simulink subsystem "Find_Catmull_Rom_Vel"  (R2023b)
settings: Solver=VariableStepAuto  StartTime=0.0  StopTime=10.0  RelTol=1e-3
settings Model: Creator=FIRSTMentor  LastModifiedBy=FIRSTMentor

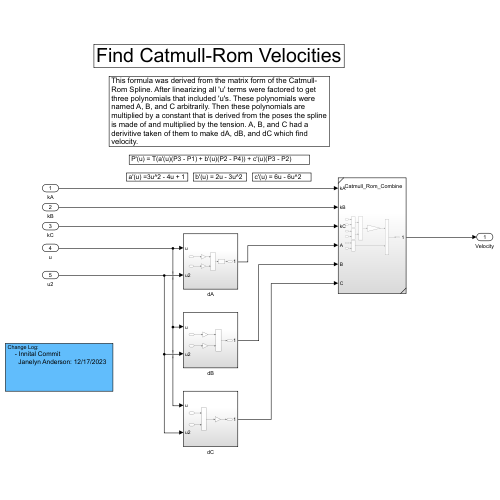
[thumbnail: Simulink's stored preview of the top-level diagram]
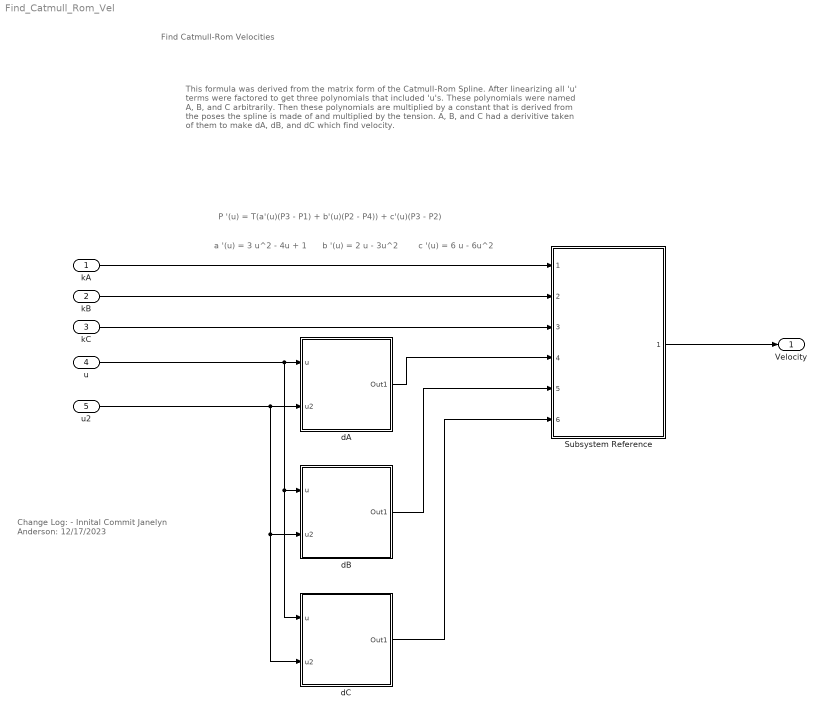
== system Find_Catmull_Rom_Vel ==
  note: Change Log:
      | - Innital Commit
      | Janelyn Anderson: 12/17/2023
  note: Find Catmull-Rom Velocities
  note: P '(u) = T(a'(u)(P3 - P1) + b'(u)(P2 - P4)) + c'(u)(P3 - P2)
  note: This formula was derived from the matrix form of the Catmull-Rom Spline. After linearizing all 'u' terms were factored to get three polynomials that included 'u's. These polynomials were named A, B, and C arbitrarily. Then these polynomials are multiplied by a constant that is derived from the poses the spline is made of and multiplied by the tension. A, B, and C had a derivitive taken of them to make dA, dB, and dC which find velocity.
  note: a '(u) = 3 u^2 - 4u + 1
  note: b '(u) = 2 u - 3u^2
  note: c '(u) = 6 u - 6u^2
  kA : Inport  PortDimensions=[1 2]
  kB : Inport  Port=2  PortDimensions=[1 2]
  kC : Inport  Port=3  PortDimensions=[1 2]
  u : Inport  Port=4  PortDimensions=1
  u2 : Inport  Port=5  PortDimensions=1
  Subsystem Reference : Subsystem  ReferencedSubsystem=Catmull_Rom_Combine
  dA : Subsystem
  dB : Subsystem
  dC : Subsystem
  Velocity : Outport
  wires:
  kA/1 -> Subsystem Reference/1
  dA/1(Out1) -> Subsystem Reference/4
  kC/1 -> Subsystem Reference/3
  kB/1 -> Subsystem Reference/2
  Subsystem Reference/1 -> Velocity/1
  dC/1(Out1) -> Subsystem Reference/6
  u/1 -> dC/1(u), dB/1(u), dA/1(u)
  dB/1(Out1) -> Subsystem Reference/5
  u2/1 -> dC/2(u2), dB/2(u2), dA/2(u2)

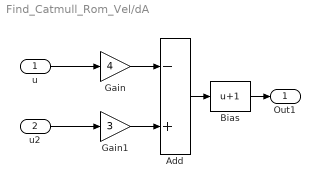
== system Find_Catmull_Rom_Vel/dA ==
  u : Inport
  u2 : Inport  Port=2
  Add : Sum  Inputs=-+
  Bias : Bias  Bias=1  SaturateOnIntegerOverflow=off
  Gain : Gain  Gain=4
  Gain1 : Gain  Gain=3
  Out1 : Outport
  wires:
  Gain1/1 -> Add/2
  Add/1 -> Bias/1
  Gain/1 -> Add/1
  Bias/1 -> Out1/1
  u/1 -> Gain/1
  u2/1 -> Gain1/1

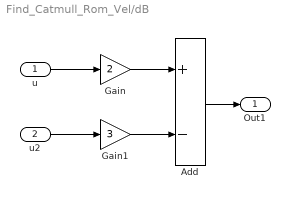
== system Find_Catmull_Rom_Vel/dB ==
  u : Inport
  u2 : Inport  Port=2
  Add : Sum  Inputs=+-
  Gain : Gain  Gain=2
  Gain1 : Gain  Gain=3
  Out1 : Outport
  wires:
  Add/1 -> Out1/1
  Gain1/1 -> Add/2
  Gain/1 -> Add/1
  u/1 -> Gain/1
  u2/1 -> Gain1/1

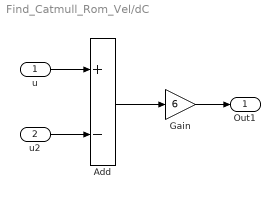
== system Find_Catmull_Rom_Vel/dC ==
  u : Inport
  u2 : Inport  Port=2
  Add : Sum  Inputs=+-
  Gain : Gain  Gain=6
  Out1 : Outport
  wires:
  Add/1 -> Gain/1
  u2/1 -> Add/2
  u/1 -> Add/1
  Gain/1 -> Out1/1
